simulink model "Pd_controller"  (R2019b)
settings: Solver=VariableStepAuto  StartTime=0.0  StopTime=20  FixedStep=.001  MaxStep=.1  RelTol=1e-3
settings Model: Creator=imi  LastModifiedBy=Ali Alaei
settings DataIOCC: ReturnWorkspaceOutputs=off
settings DebuggingCC: ArithmeticOperatorsInVariantConditions=warning
settings SFSimCC: SimUseLocalCustomCode=off  CustomCodeUndefinedFunction=UseInterfaceOnly
settings RTWCC: RTWUseLocalCustomCode=off
settings CodeAppCC: StateflowObjectComments=on

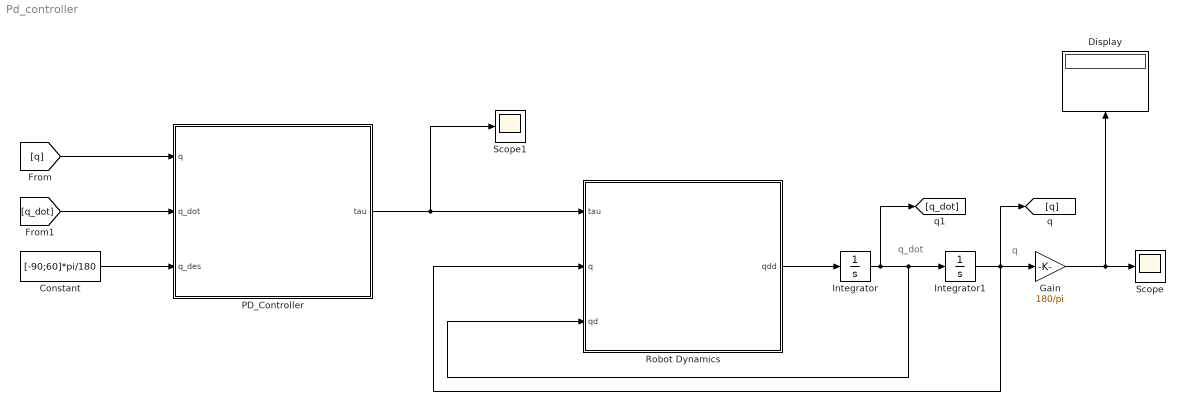
== system Pd_controller ==
  note: q
  note: q_dot
  Constant : Constant  Value=[-90;60]*pi/180
  Display : Display
  Gain : Gain  Gain=180/pi
  Integrator : Integrator  InitialCondition=zeros(2,1)
  Integrator1 : Integrator  InitialCondition=[45;95]*pi/180*0
  PD_Controller : MATLAB Function  TreatAsAtomicUnit=on
  Robot Dynamics : MATLAB Function  TreatAsAtomicUnit=on
  Scope : Scope
  Scope1 : Scope
  wires:
  Integrator/1 -> [q_dot], Robot Dynamics/3(qd), Integrator1/1
  Robot Dynamics/1(qdd) -> Integrator/1
  Integrator1/1 -> [q], Gain/1, Robot Dynamics/2(q)
  PD_Controller/1(tau) -> Scope1/1, Robot Dynamics/1(tau)
  Gain/1 -> Scope/1, Display/1
  Constant/1 -> PD_Controller/3(q_des)
  [q] -> PD_Controller/1(q)
  [q_dot] -> PD_Controller/2(q_dot)

== matlab function Pd_controller/PD_Controller ==
  data: q input; q_dot input; tau output; q_des input
function tau = fcn(q,q_dot,q_des)

Kp=eye(2);
Kd=2*eye(2);
q1=q(1);
q2=q(2);

q1d=q_dot(1);
q2d=q_dot(2);



m1=2;
m2=1.4;

I1=.5;
I2=.1;

l1=.8;
l2=.8;

lc1=.4;
lc2=.4;


g=9.81;



d11=m1*lc1^2+I1+I2+m2*(l1^2+lc2^2+2*l1*lc2*cos(q2));
d12=m2*lc2^2+I2+m2*l2*lc2*cos(q2);
d21=m2*lc2^2+I2+m2*l2*lc2*cos(q2);
d22=m2*lc2^2+I2;

c11=-m2*l1*lc2*sin(q2)*q2d;
c12=-m2*l1*lc2*sin(q2)*(q1d+q2d);
c21=m2*l1*lc2*sin(q2)*q1d;
c22=0;

g11=m1*lc1*g*cos(q1)+m2*g*(lc2*cos(q1+q2)+l1*cos(q1));
g21=m2*lc2*g*cos(q1+q2);

M=[d11,d12;d21,d22];
C=[c11 c12;c21 c22];
G=[g11;g21];




tau=C*q_dot+G-Kp*(q-q_des)-Kd*q_dot;

== matlab function Pd_controller/Robot Dynamics ==
  data: tau input; q input; qdd output; qd input
function qdd = fcn(tau,q,qd)

q1=q(1);
q2=q(2);

q1d=qd(1);
q2d=qd(2);



m1=2;
m2=1.4;

I1=.5;
I2=.1;

l1=.8;
l2=.8;

lc1=.4;
lc2=.4;


g=9.81;



d11=m1*lc1^2+I1+I2+m2*(l1^2+lc2^2+2*l1*lc2*cos(q2));
d12=m2*lc2^2+I2+m2*l2*lc2*cos(q2);
d21=m2*lc2^2+I2+m2*l2*lc2*cos(q2);
d22=m2*lc2^2+I2;

c11=-m2*l1*lc2*sin(q2)*q2d;
c12=-m2*l1*lc2*sin(q2)*(q1d+q2d);
c21=m2*l1*lc2*sin(q2)*q1d;
c22=0;

g11=m1*lc1*g*cos(q1)+m2*g*(lc2*cos(q1+q2)+l1*cos(q1));
g21=m2*lc2*g*cos(q1+q2);

M=[d11,d12;d21,d22];
C=[c11 c12;c21 c22];
G=[g11;g21];


qdd=pinv(M)*(tau-C*qd-G);
